simulink model "VirtualMotoTemplate"  (R2025b)
settings: Solver=daessc  StartTime=0  StopTime=2474  FixedStep=.001  RelTol=1e-2  EnableMultiTasking=on
StopFcn:
  | %toc
undefined symbols (not defined in the file): AccelOvrCmd, CtrlTcuInitGear, DecelOvrCmd, Disabled, DriverPreviewDist, EnblAccelOvr, EnblDecelCmd, EnblSteerCmd, EnvAbsPrs, EnvAirTemp, EnvGrvty, EnvNomFrictionScaling, EnvNominalGrade, EnvWindVelX, EnvWindVelY, EnvWindVelZ, FTP75, MotoFrmInert, MotoFrmLngth, MotoFrmMass, MotoLowrFrntFrkMass, MotoRearArmLngth, MotoRearArmMass, MotoUpprFrntFrkMass, RiderLkAhdPtDstGain, RiderMass, ScnAccTbl, ScnBrkTbl, ScnCRMaxLatAccel, ScnCRRadius, ScnDLCGateLongPos, ScnDLCLatRef, ScnDLCLatRefOffset, ScnDLCLongRefBpt, ScnDLCLongRefStartPos, ScnDLCVehicleWidth, ScnFHCounterDwellTime, ScnFHInitialDwellTime, ScnFHReturnTime, ScnFHRollRateZeroCross, ScnFHSteerAmp, ScnFHSteerSpeed, ScnISHandwheelRate, ScnISMaxHandwheelAng, ScnISMaxLatAccel, ScnISSteerHoldTime, ScnLongPosBpts, ScnLongVelRef, ScnOvalTrackl, ScnOvalTrackpdst, ScnOvalTrackr, ScnSDDwellTime, ScnSDSteerAmp, ScnSDSteerFreq, ScnSSFinalFreq, ScnSSSteerAmp, ScnSSSweepTime, ScnStartTime, ScnStrgAngTbl, ScnStrgTrqTbl ... (+10)
libraries: simulink x16, vehdynlibscenariocommon x9, sm_lib x6, autolibshared x4, nesl_utility x4, vehdynlibviscommon x3, sim3dgroundtruthsensorlib x2, vehdynlibdriver x2, sharedtransform x1, autolibutils x1, sim3dautolib x1, sim3dlib x1
(part 6 of 6)

== system VirtualMotoTemplate/Rider Commands/Rider Commands/Roll angle control/Rider Steering Control/Rider Steering/Target trajectory driving - Look ahead point/LAPview/Origin&Env/Ground ==
  Spline : sm_lib/Curves and Surfaces/Spline  DataPoints=trackData'+[0 0 0.001]  DataPointsUnits=m  EndConditionType=Natural  GraphicType=FromGeometry  MarkerShape=Sphere  MarkerSize=10  GraphicVisPropType=SimpleVisualProperties  GraphicDiffuseColor=[0.2 1.0 1.0]  GraphicOpacity=1.0  GraphicSpecularColor=[0.5 0.5 0.5 1.0]  GraphicAmbientColor=[0.15 0.15 0.15 1.0]  GraphicEmissiveColor=[0.0 0.0 0.0 1.0]  GraphicShininess=75
  Weld Joint : sm_lib/Joints/Weld Joint  JointMode=Normal  CompositeWrenchDir=FollowerOnBase  CompositeWrenchFrame=BaseFrame  SenseConstraintForce=off  SenseConstraintTorque=off  SenseTotalForce=off  SenseTotalTorque=off
  B : PMIOPort  Side=Left
  connections:
  Weld Joint/LConn1 -- B/RConn1
  Spline/LConn1 -- Weld Joint/RConn1

== matlab function VirtualMotoTemplate/Rider Commands/Rider Commands/Roll angle control/Rider Steering Control/Rider Steering/Target trajectory driving - Look ahead point/LateralDeviationDeriver ==
  settings: updateMethod=DISCRETE  sampleTime=1e-2
  data: current_x input; mindist_out output; current_y input; VehicleYaw input; trackData parameter
%%%%%%%%%%%%%%%%%%%%%%%%%%%%%%%%%%%%%%%%%%%%%%%%%%%%%%%%%%%%%%%%%%%%%%%%%%%
%                      Lateral Deviation Deriver
%
% This script derive lateral distance between lookahead point and target
% path
%%%%%%%%%%%%%%%%%%%%%%%%%%%%%%%%%%%%%%%%%%%%%%%%%%%%%%%%%%%%%%%%%%%%%%%%%%%
function mindist_out =  LateralDeviationDeriver(current_x, current_y, VehicleYaw, trackData)

mindist_out =  LateralDeviationDeriver_s(trackData, current_x, current_y, VehicleYaw);

if isnan(mindist_out)
    disp('nan!!!');
end

end

function mindist_out =  LateralDeviationDeriver_s(Target, current_x, current_y, VehicleYaw)

coder.allowpcode('plain');

% Tick = 0.1;
% 
%-------------------------------------------------------------------------%
% TARGET PATH
%-------------------------------------------------------------------------%
Target_X = Target(1,:);
Target_Y = Target(2,:);

% % interpolate
% tmp_elem     = 1:length(tmp_Target_X);
% tmp_elem_int = 1:Tick:length(tmp_Target_X);
% Target_X = interp1(tmp_elem, tmp_Target_X, tmp_elem_int,'spline');
% Target_Y = interp1(tmp_elem, tmp_Target_Y, tmp_elem_int,'spline');

%-------------------------------------------------------------------------%
% ROTATION
%-------------------------------------------------------------------------%
% rotation matrix
rotmat_yaw = [cos(VehicleYaw), -sin(VehicleYaw); sin(VehicleYaw), cos(VehicleYaw)];

% rotate target path
tmp_Target  = transpose(rotmat_yaw) * [Target_X; Target_Y];
Target_Xrot = tmp_Target(1,:);
Target_Yrot = tmp_Target(2,:);

% rotate current position
tmp_current  = transpose(rotmat_yaw) * [current_x; current_y];
current_xrot = tmp_current(1,:);
current_yrot = tmp_current(2,:);

% distance between LAP and all points
dist = sqrt((current_xrot - Target_Xrot).^2 + (current_yrot - Target_Yrot).^2);

% minimum distance point
[~, col]      = find(dist == min(abs(dist)));
% point_out = Target_Xrot(col);

%
if col(end) < length(Target_Xrot)
theta = atan((Target_Yrot(col(end)+1) - Target_Yrot(col(end))) / (Target_Xrot(col(end)+1) - Target_Xrot(col(end)))); % ??????????
else
theta = atan((Target_Yrot(col(end)) - Target_Yrot(col(end)-1)) / (Target_Xrot(col(end)) - Target_Xrot(col(end)-1)));
end

% rotation matrix
rotmat = [cos(theta), -sin(theta); sin(theta), cos(theta)];

% Coordinate transformation
if col(end) < length(Target_Xrot)
ABC_XY = [Target_Xrot(col(end)), Target_Xrot(col(end)+1), current_xrot; Target_Yrot(col(end)), Target_Yrot(col(end)+1), current_yrot];
else
ABC_XY = [Target_Xrot(col(end)-1), Target_Xrot(col(end)), current_xrot; Target_Yrot(col(end)-1), Target_Yrot(col(end)), current_yrot];
end
ABC_XYrot = transpose(rotmat) * ABC_XY;

% area
A_x = ABC_XYrot(1,1);
B_x = ABC_XYrot(1,2);
C_x = ABC_XYrot(1,3);
C_y = ABC_XYrot(2,3)-ABC_XYrot(2,1);

    area_out = 0;
if A_x <= C_x && C_x <= B_x
    area_out = 0;
elseif  C_x < A_x
    area_out = -1;
elseif  B_x < C_x
    area_out = 1;
end

% area
if area_out == -1
    if col(end) ~= 1
        if Target_Xrot(col(end)) ~= Target_Xrot(col(end)-1)
            theta = atan((Target_Yrot(col(end)) - Target_Yrot(col(end)-1)) / (Target_Xrot(col(end)) - Target_Xrot(col(end)-1)));
        else
            theta = 0;
        end
rotmat = [cos(theta), -sin(theta); sin(theta), cos(theta)];

ABC_XY = [Target_Xrot(col(end)-1), Target_Xrot(col(end)), current_xrot; Target_Yrot(col(end)-1), Target_Yrot(col(end)), current_yrot];
    else
        if Target_Xrot(col(end)) ~= Target_Xrot(end)
            theta = atan((Target_Yrot(col(end)) - Target_Yrot(end)) / (Target_Xrot(col(end)) - Target_Xrot(end)));
        else
            theta = 0;
        end
rotmat = [cos(theta), -sin(theta); sin(theta), cos(theta)];

ABC_XY = [Target_Xrot(end), Target_Xrot(col(end)), current_xrot; Target_Yrot(end), Target_Yrot(col(end)), current_yrot];
    end
    
ABC_XYrot = transpose(rotmat) * ABC_XY;

% A.y = ABC_XYrot(2,1);
% B.y = ABC_XYrot(2,2);
C_y = ABC_XYrot(2,3)-ABC_XYrot(2,1);
end

% minimum distance
mindist_out = C_y;
end

== matlab function VirtualMotoTemplate/Visualization/Excessive Roll Angle Detection ==
  data: phi input; stopSim output
function stopSim = phiStop(phi)
%#codegen

% Initialize output
stopSim = false;

% Check the condition
rollLim = pi/3;
if abs(phi)>=rollLim
    % Display a warning message    
    warning(message('vdynblks:vehdynErrMsg:excessivePhi',num2str(rad2deg(rollLim))));
    % Set output to indicate a warning has been triggered
    stopSim = true;
end
